simulink model "strojenie_reg_pomocniczego"  (R2018b)
settings: Solver=FixedStepAuto  StartTime=0.0  StopTime=T_symulacji  FixedStep=t_krok  RelTol=1e-3
values from neighbouring files (symbols this model uses):
  k_p = nastawy_p(1)    [opt_str_reg_pom.m]    (also in reg_pom_P.m = k_p0; reg_pom_PD.m = k_p0; reg_pom_PI.m = k_p0; reg_pom_PID.m = k_p0)
  Td_p = nastawy_p(3)    [opt_str_reg_pom.m]    (also in reg_pom_P.m = 0; reg_pom_PD.m = Td_p0; reg_pom_PI.m = 0; reg_pom_PID.m = Td_p0)
  Ti_p = nastawy_p(2)    [opt_str_reg_pom.m]    (also in reg_pom_P.m = inf; reg_pom_PD.m = inf; reg_pom_PI.m = Ti_p0; reg_pom_PID.m = Ti_p0)
undefined symbols (not defined in the file or in its folder): G_sz
libraries: simulink x1
settings Model: Creator=Admin  LastModifiedBy=Admin

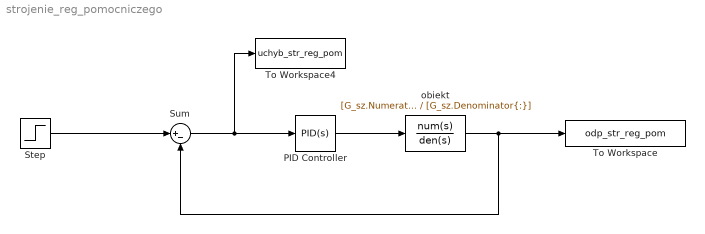
== system strojenie_reg_pomocniczego ==
  " obiekt" : TransferFcn  Numerator=[G_sz.Numerator{:}]  Denominator=[G_sz.Denominator{:}]
  PID Controller : simulink/Continuous/PID Controller  Controller=PID  Form=Ideal  TimeDomain=Continuous-time  SampleTime=-1  IntegratorMethod=Forward Euler  FilterMethod=Forward Euler  ControllerParametersSource=internal  P=k_p  I=1/Ti_p  D=Td_p  UseFilter=on  N=100  TunerSelectOption=Transfer Function Based (PID Tuner App)  InitialConditionSource=internal  InitialConditionForIntegrator=0  InitialConditionForFilter=0  DifferentiatorICPrevScaledInput=0  ExternalReset=none  TrackingMode=off  Kt=1  LimitOutput=off  UpperSaturationLimit=inf  LowerSaturationLimit=-inf  LinearizeAsGain=on  AntiWindupMode=none  Kb=1  POutMin=[]  POutMax=[]  IOutMin=[]  IOutMax=[]  DOutMin=[]  DOutMax=[]  NOutMin=[]  NOutMax=[]  SumOutMin=[]  SumOutMax=[]  SaturationOutMin=[]  SaturationOutMax=[]  PParamMin=[]  PParamMax=[]  IParamMin=[]  IParamMax=[]  DParamMin=[]  DParamMax=[]  NParamMin=[]  NParamMax=[]  KbParamMin=[]  KbParamMax=[]  KtParamMin=[]  KtParamMax=[]  KbOutMin=[]  KbOutMax=[]  KtOutMin=[]  KtOutMax=[]  IntegratorOutMin=[]  IntegratorOutMax=[]  FilterOutMin=[]  FilterOutMax=[]  SumI1OutMin=[]  SumI1OutMax=[]  SumI2OutMin=[]  SumI2OutMax=[]  SumI3OutMin=[]  SumI3OutMax=[]  SumI4OutMin=[]  SumI4OutMax=[]  SumDOutMin=[]  SumDOutMax=[]  DifferentiatorOutMin=[]  DifferentiatorOutMax=[]  FilterDiffOutCoefMin=[]  FilterDiffOutCoefMax=[]  ReciprocalOutMin=[]  ReciprocalOutMax=[]  SumDenOutMin=[]  SumDenOutMax=[]  SumNumOutMin=[]  SumNumOutMax=[]  DivideOutMin=[]  DivideOutMax=[]  IntegratorContinuousStateAttributes=''  IntegratorStateMustResolveToSignalObject=off  IntegratorRTWStateStorageClass=Auto  FilterContinuousStateAttributes=''  FilterStateMustResolveToSignalObject=off  FilterRTWStateStorageClass=Auto  ParallelPVariant=Passthrough  IdealPVariant=InternalParameters  IVariant=InternalParameters  DVariant=InternalParameters  IntegratorVariant=Continuous  SatVariant=Disabled  AWVariant=Passthrough  PCopyVariant=Disabled  TRVariant=Disabled  FdbkBlocksVariant=Forward  IdealPFdbkVariant=Disabled  SatFdbkVariant=Disabled  DerivativeFilterVariant=ContFilter  NVariant=InternalParameters  NCopyVariant=Disabled  FilterICVariant=InternalICsFilter  IntegratorICVariant=InternalICs  ExternalResetVariant=Disabled  TRSumVariant=Passthrough  SumFdbkVariant=Disabled  SumVariant=Sum_PID
  Step : Step  Time=0  SampleTime=0
  Sum : Sum  Inputs=|+-
  To Workspace : ToWorkspace  VariableName=odp_str_reg_pom  SampleTime=-1
  To Workspace4 : ToWorkspace  VariableName=uchyb_str_reg_pom  SampleTime=-1
  wires:
  " obiekt"/1 -> Sum/2, To Workspace/1
  Step/1 -> Sum/1
  Sum/1 -> PID Controller/1, To Workspace4/1
  PID Controller/1 -> " obiekt"/1
